simulink model "preprojeto2_simulink"  (R2020a)
settings: Solver=FixedStepAuto  StartTime=0.0  StopTime=3  FixedStep=0.00001  RelTol=1e-3
values from neighbouring files (symbols this model uses):
  kd = 10    [preprojeto2.m]
  ki = 20    [preprojeto2.m]
  kp = 50    [preprojeto2.m]
  tam = 0.1    [preprojeto2.m]
libraries: simulink x1
settings Model: Creator=gusta  LastModifiedBy=gusta

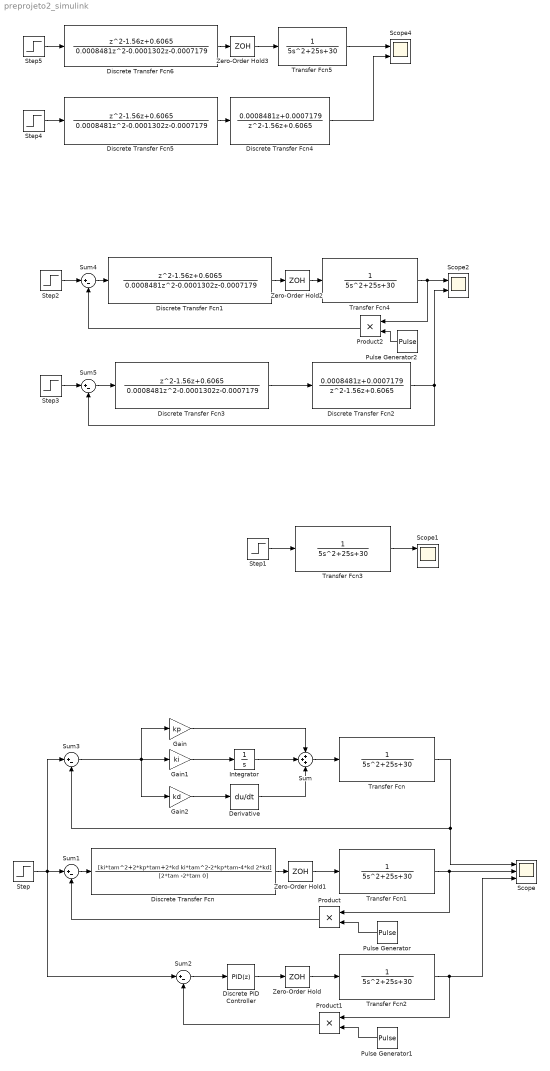
== system preprojeto2_simulink ==
  Derivative : Derivative
  Discrete Transfer Fcn : DiscreteTransferFcn  Numerator=[ki*tam^2+2*kp*tam+2*kd ki*tam^2-2*kp*tam-4*kd 2*kd]  Denominator=[2*tam -2*tam 0]  SampleTime=tam
  Discrete Transfer Fcn{1,3,5..6} (4 alike) : DiscreteTransferFcn  Numerator=[1 -1.56 0.6065]  Denominator=[0.0008481 -0.0001302 -0.0007179]  SampleTime=tam
  Discrete Transfer Fcn2 : DiscreteTransferFcn  Numerator=[0.0008481 0.0007179]  Denominator=[1 -1.56 0.6065]  SampleTime=tam
  Discrete Transfer Fcn4 : DiscreteTransferFcn  Numerator=[0.0008481 0.0007179]  Denominator=[1 -1.56 0.6065]  SampleTime=tam
  Discrete PID Controller : simulink/Continuous/PID Controller  Controller=PID  Form=Parallel  TimeDomain=Discrete-time  UseExternalTs=off  SampleTime=-1  IntegratorMethod=Forward Euler  FilterMethod=Forward Euler  ControllerParametersSource=internal  P=kp  I=ki  D=kd  UseFilter=on  N=100  TunerSelectOption=Transfer Function Based (PID Tuner App)  InitialConditionSource=internal  InitialConditionForIntegrator=0  InitialConditionForFilter=0  DifferentiatorICPrevScaledInput=0  ExternalReset=none  TrackingMode=off  Kt=1  LimitOutput=off  UpperSaturationLimit=inf  LowerSaturationLimit=-inf  LinearizeAsGain=off  AntiWindupMode=none  Kb=1  POutMin=[]  POutMax=[]  IOutMin=[]  IOutMax=[]  DOutMin=[]  DOutMax=[]  NOutMin=[]  NOutMax=[]  SumOutMin=[]  SumOutMax=[]  SaturationOutMin=[]  SaturationOutMax=[]  PParamMin=[]  PParamMax=[]  IParamMin=[]  IParamMax=[]  DParamMin=[]  DParamMax=[]  NParamMin=[]  NParamMax=[]  KbParamMin=[]  KbParamMax=[]  KtParamMin=[]  KtParamMax=[]  KbOutMin=[]  KbOutMax=[]  KtOutMin=[]  KtOutMax=[]  IntegratorOutMin=[]  IntegratorOutMax=[]  FilterOutMin=[]  FilterOutMax=[]  SumI1OutMin=[]  SumI1OutMax=[]  SumI2OutMin=[]  SumI2OutMax=[]  SumI3OutMin=[]  SumI3OutMax=[]  SumI4OutMin=[]  SumI4OutMax=[]  SumDOutMin=[]  SumDOutMax=[]  DifferentiatorOutMin=[]  DifferentiatorOutMax=[]  FilterDiffOutCoefMin=[]  FilterDiffOutCoefMax=[]  ReciprocalOutMin=[]  ReciprocalOutMax=[]  SumDenOutMin=[]  SumDenOutMax=[]  SumNumOutMin=[]  SumNumOutMax=[]  DivideOutMin=[]  DivideOutMax=[]  UdiffTsProdOutMin=[]  UdiffTsProdOutMax=[]  NTsProdOutMin=[]  NTsProdOutMax=[]  UintegralTsProdOutMin=[]  UintegralTsProdOutMax=[]  UngainTsProdOutMin=[]  UngainTsProdOutMax=[]  IntegratorContinuousStateAttributes=''  IntegratorStateMustResolveToSignalObject=off  IntegratorRTWStateStorageClass=Auto  FilterContinuousStateAttributes=''  FilterStateMustResolveToSignalObject=off  FilterRTWStateStorageClass=Auto  ParallelPVariant=InternalParameters  IdealPVariant=Disabled  IVariant=InternalParameters  DVariant=InternalParameters  IntegratorVariant=Discrete  SatVariant=Disabled  AWVariant=Passthrough  PCopyVariant=Disabled  TRVariant=Disabled  FdbkBlocksVariant=Forward  IdealPFdbkVariant=Disabled  SatFdbkVariant=Disabled  DerivativeFilterVariant=ForwardEulerFilter  NVariant=InternalParameters  NCopyVariant=Disabled  FilterICVariant=InternalICsFilter  IntegratorICVariant=InternalICs  ExternalResetVariant=Disabled  TRSumVariant=Passthrough  SumFdbkVariant=Disabled  SumVariant=Sum_PID  TsampFilterVariant=InternalTs  TsampNgainVariant=Passthrough  TsampIntegralVariant=Passthrough
  Gain : Gain  Gain=kp
  Gain1 : Gain  Gain=ki
  Gain2 : Gain  Gain=kd
  Integrator : Integrator
  Product : Product
  Product1 : Product
  Product2 : Product
  Pulse Generator : DiscretePulseGenerator  PulseType=Time based  Period=tam
  Pulse Generator1 : DiscretePulseGenerator  PulseType=Time based  Period=tam
  Pulse Generator2 : DiscretePulseGenerator  PulseType=Time based  Period=tam
  Scope : Scope  NumInputPorts=3
  Scope1 : Scope  NumInputPorts=3
  Scope2 : Scope  NumInputPorts=2
  Scope4 : Scope  NumInputPorts=2
  Step{,1..5} (6 alike) : Step  Time=0.1  SampleTime=0
  Sum : Sum  Inputs=+++
  Sum{1..5} (5 alike) : Sum  Inputs=|+-
  Transfer Fcn{,1..5} (6 alike) : TransferFcn  Denominator=[5 25 30]
  Zero-Order Hold{,1..3} (4 alike) : ZeroOrderHold  SampleTime=tam
  wires:
  Product/1 -> Sum1/2
  Step/1 -> Sum2/1, Sum3/1, Sum1/1
  Discrete PID Controller/1 -> Zero-Order Hold/1
  Gain2/1 -> Derivative/1
  Sum/1 -> Transfer Fcn/1
  Pulse Generator1/1 -> Product1/2
  Gain/1 -> Sum/1
  Integrator/1 -> Sum/2
  Zero-Order Hold/1 -> Transfer Fcn2/1
  Pulse Generator/1 -> Product/2
  Gain1/1 -> Integrator/1
  Transfer Fcn2/1 -> Product1/1, Scope/3
  Derivative/1 -> Sum/3
  Discrete Transfer Fcn/1 -> Zero-Order Hold1/1
  Product1/1 -> Sum2/2
  Sum3/1 -> Gain2/1, Gain/1, Gain1/1
  Zero-Order Hold1/1 -> Transfer Fcn1/1
  Sum1/1 -> Discrete Transfer Fcn/1
  Transfer Fcn/1 -> Sum3/2, Scope/1
  Transfer Fcn1/1 -> Product/1, Scope/2
  Sum2/1 -> Discrete PID Controller/1
  Transfer Fcn3/1 -> Scope1/1
  Step1/1 -> Transfer Fcn3/1
  Product2/1 -> Sum4/2
  Pulse Generator2/1 -> Product2/2
  Zero-Order Hold2/1 -> Transfer Fcn4/1
  Discrete Transfer Fcn1/1 -> Zero-Order Hold2/1
  Step2/1 -> Sum4/1
  Sum4/1 -> Discrete Transfer Fcn1/1
  Transfer Fcn4/1 -> Scope2/1, Product2/1
  Sum5/1 -> Discrete Transfer Fcn3/1
  Discrete Transfer Fcn3/1 -> Discrete Transfer Fcn2/1
  Step3/1 -> Sum5/1
  Discrete Transfer Fcn2/1 -> Sum5/2, Scope2/2
  Step4/1 -> Discrete Transfer Fcn5/1
  Discrete Transfer Fcn5/1 -> Discrete Transfer Fcn4/1
  Discrete Transfer Fcn4/1 -> Scope4/2
  Step5/1 -> Discrete Transfer Fcn6/1
  Discrete Transfer Fcn6/1 -> Zero-Order Hold3/1
  Zero-Order Hold3/1 -> Transfer Fcn5/1
  Transfer Fcn5/1 -> Scope4/1
